simulink model "inv_120_R"  (R2018a)
settings: Solver=FixedStepDiscrete  StartTime=0.0  StopTime=0.5  FixedStep=(1/3)*(10^(-7))  RelTol=1e-3
libraries: powerlib x15, powerlib_meascontrol x3
settings Model: Creator=KUNAL  LastModifiedBy=KUNAL

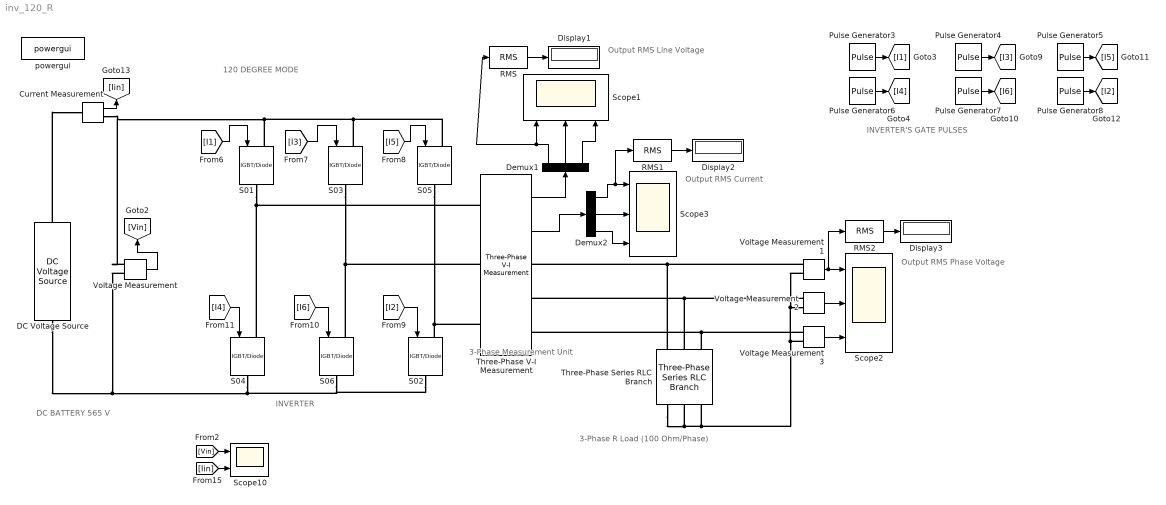
== system inv_120_R ==
  note: INVERTER'S GATE PULSES
  note: INVERTER
  note: 120 DEGREE MODE
  note: 3-Phase R Load (100 Ohm/Phase)
  note: 3-Phase Measurement Unit
  note: Output RMS Current
  note: Output RMS Line Voltage
  note: Output RMS Phase Voltage
  note: DC BATTERY
      | 565 V
  Current Measurement : powerlib/Measurements/Current Measurement  PhasorSimulation=off  OutputType=Complex  PSBequivalent=0
  DC Voltage Source : powerlib/Electrical Sources/DC Voltage Source  Amplitude=565  Measurements=None
  Demux1 : Demux  Outputs=3
  Demux2 : Demux  Outputs=3
  Display1 : Display
  Display2 : Display
  Display3 : Display
  Pulse Generator3 : DiscretePulseGenerator  PulseType=Time based  Period=0.02  PulseWidth=100/3
  Pulse Generator4 : DiscretePulseGenerator  PulseType=Time based  Period=0.02  PulseWidth=100/3  PhaseDelay=(120*0.02)/360
  Pulse Generator5 : DiscretePulseGenerator  PulseType=Time based  Period=0.02  PulseWidth=100/3  PhaseDelay=(240*0.02)/360
  Pulse Generator6 : DiscretePulseGenerator  PulseType=Time based  Period=0.02  PulseWidth=100/3  PhaseDelay=(180*0.02)/360
  Pulse Generator7 : DiscretePulseGenerator  PulseType=Time based  Period=0.02  PulseWidth=100/3  PhaseDelay=((120+180)*0.02)/360
  Pulse Generator8 : DiscretePulseGenerator  PulseType=Time based  Period=0.02  PulseWidth=100/3  PhaseDelay=((240+180)*0.02)/360
  RMS : powerlib_meascontrol/Measurements/RMS  TrueRMS=on  Freq=50  RMSInit=0  Ts=(1/3)*(10^(-7))
  RMS1 : powerlib_meascontrol/Measurements/RMS  TrueRMS=on  Freq=50  RMSInit=0  Ts=(1/3)*(10^(-7))
  RMS2 : powerlib_meascontrol/Measurements/RMS  TrueRMS=on  Freq=50  RMSInit=0  Ts=(1/3)*(10^(-7))
  S01 : powerlib/Power Electronics/IGBT//Diode  Ron=1e-3  Rs=1e5  Cs=inf  Measurements=off
  S02 : powerlib/Power Electronics/IGBT//Diode  Ron=1e-3  Rs=1e5  Cs=inf  Measurements=off
  S03 : powerlib/Power Electronics/IGBT//Diode  Ron=1e-3  Rs=1e5  Cs=inf  Measurements=off
  S04 : powerlib/Power Electronics/IGBT//Diode  Ron=1e-3  Rs=1e5  Cs=inf  Measurements=off
  S05 : powerlib/Power Electronics/IGBT//Diode  Ron=1e-3  Rs=1e5  Cs=inf  Measurements=off
  S06 : powerlib/Power Electronics/IGBT//Diode  Ron=1e-3  Rs=1e5  Cs=inf  Measurements=off
  Scope1 : Scope  NumInputPorts=3
  Scope10 : Scope  NumInputPorts=2
  Scope2 : Scope  NumInputPorts=3
  Scope3 : Scope  NumInputPorts=3
  Three-Phase Series RLC Branch : powerlib/Elements/Three-Phase Series RLC Branch  LConnTagsString=A|B|C  RConnTagsString=A|B|C  BranchType=R  Resistance=10  Inductance=0  Capacitance=0  Measurements=Branch voltages
  Three-Phase V-I Measurement : powerlib/Measurements/Three-Phase V-I Measurement  VoltageMeasurement=phase-to-phase  SetLabelV=off  LabelV=Vabc  Vpu=off  VpuLL=off  CurrentMeasurement=yes  SetLabelI=off  LabelI=Iabc  Ipu=off  Pbase=100e6  Vbase=500e3  OutputType=Complex  PhasorSimulation=off  PSBequivalent=0
  Voltage Measurement{,1..3} (4 alike) : powerlib/Measurements/Voltage Measurement  PhasorSimulation=off  OutputType=Complex  PSBequivalent=0
  powergui : powerlib/powergui  Priority=1  SimulationMode=Discrete  SampleTime=50e-6  frequency=60  Iterations=50  frequencyindice=0  Pbase=100e6  ErrMax=1e-4  UnitsV=kV  UnitsW=MW  buscounter=0  FunctionMessages=off  echomessages=off  EnableUseOfTLC=off  CurrentSourceSwitches=off  DisableSnubberDevices=off  DisableRonSwitches=off  DisableVfSwitches=off  DisplayEquations=off  SolverType=Tustin/Backward Euler (TBE)  Interpol=off  ExternalGateDelay=off  methode=off  Ts=100  x0status=blocks  SPID=off  SwTol=0  HookPort=off  RestoreLinks=warning  ResistiveCurrentMeasurement=off  Frange=[0:2:500]  Ylog=off  Xlog=on  ShowGrid=off  save=off  variable=ZData  structure=ScopeData  ZoomFFT=off  StartTime=0.0  cycles=1  DisplayStyle=1  fundamental=60  FreqAxis=off  MaxFrequency=1000  frequencyindicesteady=1  RmsSteady=1  display=off
  wires:
  [I4] -> S04/1
  [I3] -> S03/1
  Voltage Measurement/1 -> [Vin]
  Pulse Generator7/1 -> [I6]
  Pulse Generator5/1 -> [I5]
  Pulse Generator6/1 -> [I4]
  [I2] -> S02/1
  Pulse Generator8/1 -> [I2]
  Pulse Generator3/1 -> [I1]
  Pulse Generator4/1 -> [I3]
  [I6] -> S06/1
  [I5] -> S05/1
  Current Measurement/1 -> [Iin]
  [I1] -> S01/1
  Demux1/1 -> RMS/1, Scope1/1
  Demux1/2 -> Scope1/2
  Three-Phase V-I Measurement/1 -> Demux1/1
  Demux1/3 -> Scope1/3
  Voltage Measurement2/1 -> Scope2/2
  Voltage Measurement3/1 -> Scope2/3
  Three-Phase V-I Measurement/2 -> Demux2/1
  Demux2/2 -> Scope3/2
  Demux2/3 -> Scope3/3
  RMS/1 -> Display1/1
  RMS1/1 -> Display2/1
  Demux2/1 -> RMS1/1, Scope3/1
  RMS2/1 -> Display3/1
  Voltage Measurement1/1 -> Scope2/1, RMS2/1
  [Iin] -> Scope10/2
  [Vin] -> Scope10/1
  connections:
  S03/LConn1 -- S05/LConn1 -- S01/LConn1 -- Voltage Measurement/LConn1 -- Current Measurement/RConn1
  S01/RConn1 -- Three-Phase V-I Measurement/LConn1 -- S04/LConn1
  Voltage Measurement/LConn2 -- DC Voltage Source/LConn1 -- S06/RConn1 -- S02/RConn1 -- S04/RConn1
  DC Voltage Source/RConn1 -- Current Measurement/LConn1
  S05/RConn1 -- Three-Phase V-I Measurement/LConn3 -- S02/LConn1
  S03/RConn1 -- Three-Phase V-I Measurement/LConn2 -- S06/LConn1
  Voltage Measurement3/LConn2 -- Voltage Measurement1/LConn2 -- Voltage Measurement2/LConn2 -- Three-Phase Series RLC Branch/LConn1 -- Three-Phase Series RLC Branch/LConn2 -- Three-Phase Series RLC Branch/LConn3
  Voltage Measurement3/LConn1 -- Three-Phase V-I Measurement/RConn3 -- Three-Phase Series RLC Branch/RConn3
  Voltage Measurement1/LConn1 -- Three-Phase V-I Measurement/RConn1 -- Three-Phase Series RLC Branch/RConn1
  Voltage Measurement2/LConn1 -- Three-Phase V-I Measurement/RConn2 -- Three-Phase Series RLC Branch/RConn2
